simulink model "Model3"  (R2015b)
settings: Solver=ode45  StartTime=0.0  StopTime=3  RelTol=1e-6
undefined symbols (not defined in the file): B_f, B_w, g, J_f, J_w, l_f, l_w, m_f, m_w
settings Model: Creator=USUARIO  LastModifiedBy=USUARIO
settings DataIOCC: LimitDataPoints=off  SaveFormat=Array
settings DebuggingCC: SolverPrmCheckMsg=warning
settings HardwareCC: ProdBitPerPointer=32  ProdLargestAtomicFloat=None  ProdIntDivRoundTo=Undefined  ProdEndianess=Unspecified  ProdWordSize=32  ProdHWDeviceType=32-bit Generic
settings GRTTargetCC: GeneratePreprocessorConditionals=Disable all
settings ConfigComp: CovModelRefEnable=Off  CovSFcnEnable=off

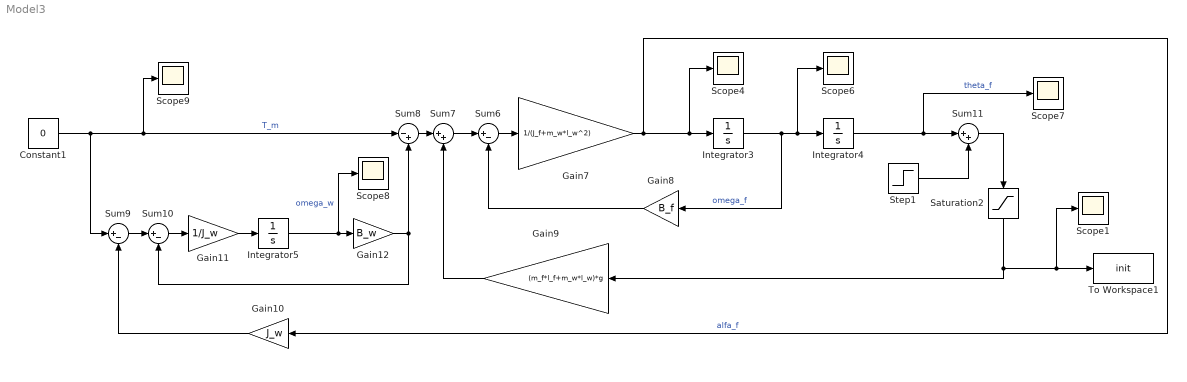
== system Model3 ==
  Constant1 : Constant  Value=0
  Gain10 : Gain  Gain=J_w
  Gain11 : Gain  Gain=1/J_w
  Gain12 : Gain  Gain=B_w
  Gain7 : Gain  Gain=1/(J_f+m_w*l_w^2)
  Gain8 : Gain  Gain=B_f
  Gain9 : Gain  Gain=(m_f*l_f+m_w*l_w)*g
  Integrator3 : Integrator
  Integrator4 : Integrator
  Integrator5 : Integrator
  Saturation2 : Saturate  UpperLimit=0.85  LowerLimit=-0.72
  Scope{1,4,6..9} (6 alike) : Scope
  Step1 : Step  Time=0.001  Before=-0.0002  After=0  SampleTime=0
  Sum10 : Sum  Inputs=|+-
  Sum11 : Sum  Inputs=|++
  Sum6 : Sum  Inputs=|+-
  Sum7 : Sum  Inputs=|++
  Sum8 : Sum  Inputs=|-+
  Sum9 : Sum  Inputs=|+-
  To Workspace1 : ToWorkspace  VariableName=init  SaveFormat=Timeseries  SampleTime=-1
  wires:
  Gain7/1 -> Gain10/1, Scope4/1, Integrator3/1  "alfa_f"
  Integrator3/1 -> Gain8/1, Scope6/1, Integrator4/1  "omega_f"
  Sum6/1 -> Gain7/1
  Sum7/1 -> Sum6/1
  Gain8/1 -> Sum6/2
  Gain9/1 -> Sum7/2
  Sum8/1 -> Sum7/1
  Sum10/1 -> Gain11/1
  Gain11/1 -> Integrator5/1
  Gain10/1 -> Sum9/2
  Sum9/1 -> Sum10/1
  Integrator5/1 -> Scope8/1, Gain12/1  "omega_w"
  Gain12/1 -> Sum10/2, Sum8/2
  Constant1/1 -> Sum9/1, Scope9/1, Sum8/1  "T_m"
  Integrator4/1 -> Scope7/1, Sum11/1  "theta_f"
  Step1/1 -> Sum11/2
  Sum11/1 -> Saturation2/1
  Saturation2/1 -> Gain9/1, Scope1/1, To Workspace1/1
